simulink model "Robot_subsistema"  (R2019a)
settings: Solver=VariableStepAuto  StartTime=0.0  StopTime=10.0  RelTol=1e-3
undefined symbols (not defined in the file): DiscIntNeverNeededParam
settings Model: Creator=mrblissfulgrin  LastModifiedBy=mrblissfulgrin

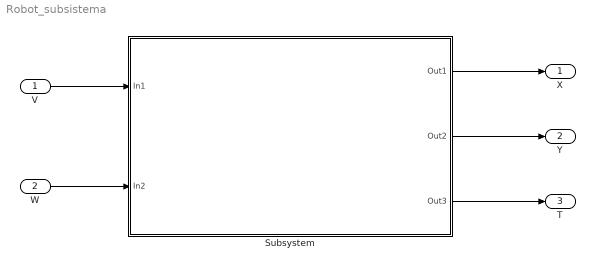
== system Robot_subsistema ==
  V : Inport
  W : Inport  Port=2
  Subsystem : Subsystem
  X : Outport
  Y : Outport  Port=2
  T : Outport  Port=3
  wires:
  V/1 -> Subsystem/1(In1)
  W/1 -> Subsystem/2(In2)
  Subsystem/1(Out1) -> X/1
  Subsystem/2(Out2) -> Y/1
  Subsystem/3(Out3) -> T/1

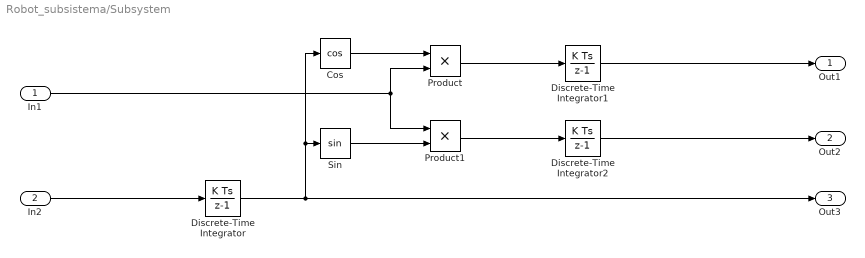
== system Robot_subsistema/Subsystem ==
  In1 : Inport
  In2 : Inport  Port=2
  Cos : Trigonometry  Operator=cos
  Discrete-Time Integrator : DiscreteIntegrator  InitialCondition=30*pi/180  SampleTime=0.01  ICPrevOutput=DiscIntNeverNeededParam  ICPrevScaledInput=DiscIntNeverNeededParam
  Discrete-Time Integrator1 : DiscreteIntegrator  SampleTime=0.01  ICPrevOutput=DiscIntNeverNeededParam  ICPrevScaledInput=DiscIntNeverNeededParam
  Discrete-Time Integrator2 : DiscreteIntegrator  SampleTime=0.01  ICPrevOutput=DiscIntNeverNeededParam  ICPrevScaledInput=DiscIntNeverNeededParam
  Product : Product
  Product1 : Product
  Sin : Trigonometry
  Out1 : Outport
  Out2 : Outport  Port=2
  Out3 : Outport  Port=3
  wires:
  Discrete-Time Integrator2/1 -> Out2/1
  Product1/1 -> Discrete-Time Integrator2/1
  Cos/1 -> Product/1
  Sin/1 -> Product1/2
  In2/1 -> Discrete-Time Integrator/1
  Discrete-Time Integrator1/1 -> Out1/1
  Product/1 -> Discrete-Time Integrator1/1
  In1/1 -> Product/2, Product1/1
  Discrete-Time Integrator/1 -> Out3/1, Sin/1, Cos/1
